simulink model "Md57StEnCtrl"  (R2018b)
settings: Solver=FixedStepDiscrete  StartTime=0.0  StopTime=10.0  FixedStep=0.01  RelTol=1e-3
undefined symbols (not defined in the file or in its folder): data, KeSMSuFirstRwStFwdBkwdPosDelta_Val, KeSMSw4SSecRwLtStLgrstUpwdDnwdOpenPos1_Val, PassStBkReclnEn_Clear, PassStBkReclnEn_Set, PassStFldEn_Clear, PassStFldEn_Set, PassStFwdBkwdEn_Clear, PassStFwdBkwdEn_Set, SecRwRtStBkReclnEn_Clear, SecRwRtStBkReclnEn_Set, SecRwRtStFwdBkwdEn_Clear, SecRwRtStFwdBkwdEn_Set, SecRwRtStLgrstInwdOtwdEn_Clear, SecRwRtStLgrstInwdOtwdEn_Set, SecRwRtStLgrstUpwdDnwdEn_Clear, SecRwRtStLgrstUpwdDnwdEn_Set, ThdRwLtStBkReclnEn_Clear, ThdRwLtStBkReclnEn_Set, ThdRwLtStFwdBkwdEn_Clear, ThdRwLtStFwdBkwdEn_Set, ThdRwRtStBkReclnEn_Clear, ThdRwRtStBkReclnEn_Set, ThdRwRtStFwdBkwdEn_Clear, ThdRwRtStFwdBkwdEn_Set, ZeroREn_Clear, ZeroREn_Set
libraries: simulink x1
(part 1 of 2)
settings Model: Creator=sn2xws  LastModifiedBy=sn2xws
settings Model: ModifiedHistory=|
  | 2024.10.15 V3.0.0 新增模式Md57
  | 2024.11.18 V3.0.1 CR946373
settings DataIOCC: SaveFormat=StructureWithTime
settings OptimizationCC: DefaultParameterBehavior=Inlined  EnhancedBackFolding=on  PassReuseOutputArgsAs=Individual arguments  ZeroExternalMemoryAtStartup=off  ZeroInternalMemoryAtStartup=off  OptimizeBlockOrder=speed  DifferentSizesBufferReuse=on  OptimizationCustomize=off
settings DebuggingCC: ParameterTunabilityLossMsg=error
settings SFSimCC: MATLABDynamicMemAlloc=off
settings RTWCC: SystemTargetFile=autosar.tlc  GenCodeOnly=on  TemplateMakefile=ert_default_tmf  Description=AUTOSAR  GenerateReport=on  IncludeHyperlinkInReport=on  LaunchReport=on  GenerateTraceInfo=on  GenerateTraceReport=on  GenerateTraceReportSl=on  GenerateTraceReportSf=on  GenerateTraceReportEml=on
settings CodeAppCC: ForceParamTrailComments=on  IgnoreCustomStorageClasses=off  OperatorAnnotations=on  SimulinkDataObjDesc=on  SFDataObjDesc=on  InsertBlockDesc=on
settings STFCustomTargetCC: TargetLangStandard=C99 (ISO)  MultiwordLength=256  ParMdlRefBuildCompliant=on  CompOptLevelCompliant=on  IncludeMdlTerminateFcn=off  CombineOutputUpdateFcns=on  SuppressErrorStatus=on  ERTCustomFileBanners=on  SupportNonFinite=off  SupportComplex=off  SupportContinuousTime=off  SupportNonInlinedSFcns=off  RemoveResetFunc=on  MATLABClassNameForMDSCustomization=Simulink.SoftwareTarget.ERTCustomization  AutosarCompliant=on  UseToolchainInfoCompliant=on  LookupTableObjectStructAxisOrder=2,1,3,4,...  LUTObjectStructOrderEvenSpacing=Size,Table,Breakpoints  SystemTargetFile=autosar.tlc
settings ERTTargetCC: TargetLangStandard=C99 (ISO)  ConcurrentExecutionCompliant=off  IncludeMdlTerminateFcn=off  SuppressErrorStatus=on  SupportNonFinite=off  SupportComplex=off  ModelStepFunctionPrototypeControlCompliant=off  CPPClassGenCompliant=off  AutosarCompliant=on  LookupTableObjectStructAxisOrder=2,1,3,4,...  LUTObjectStructOrderEvenSpacing=Size,Table,Breakpoints  InlinedParameterPlacement=NonHierarchical  ERTCustomFileTemplate=example_file_process.tlc  ERTFilePackagingFormat=Compact

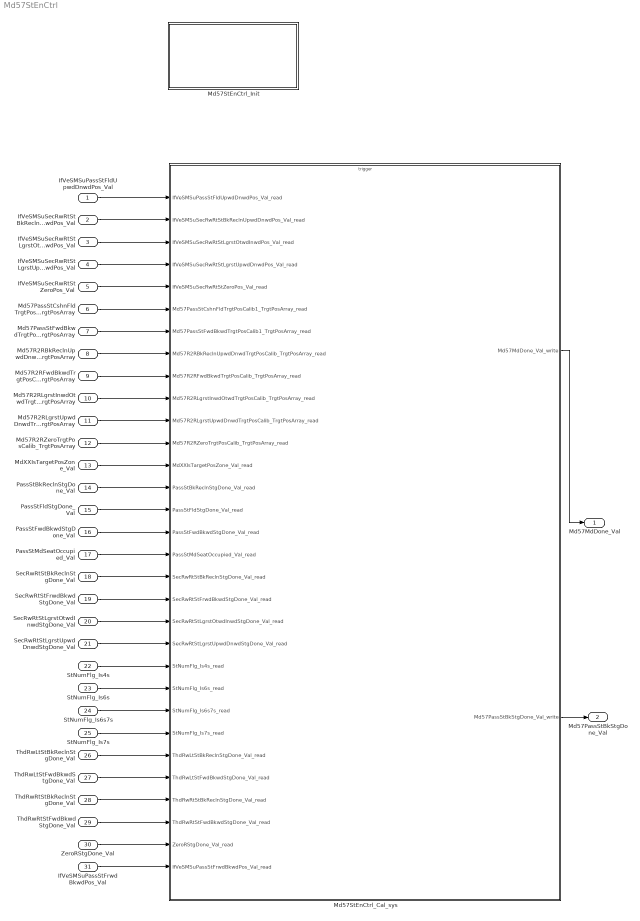
== system Md57StEnCtrl ==
  IfVeSMSuPassStFldUpwdDnwdPos_Val : Inport  OutDataTypeStr=uint16  PortDimensions=1
  IfVeSMSuSecRwRtStBkReclnUpwdDnwdPos_Val : Inport  Port=2  OutDataTypeStr=uint16  PortDimensions=1
  IfVeSMSuSecRwRtStLgrstOtwdInwdPos_Val : Inport  Port=3  OutDataTypeStr=uint16  PortDimensions=1
  IfVeSMSuSecRwRtStLgrstUpwdDnwdPos_Val : Inport  Port=4  OutDataTypeStr=uint16  PortDimensions=1
  IfVeSMSuSecRwRtStZeroPos_Val : Inport  Port=5  OutDataTypeStr=uint16  PortDimensions=1
  Md57PassStCshnFldTrgtPosCalib1_TrgtPosArray : Inport  Description=|  Port=6  OutDataTypeStr=uint16  PortDimensions=3
      | 0:Pos
      | 1:Max
      | 2:Min
  Md57PassStFwdBkwdTrgtPosCalib1_TrgtPosArray : Inport  Description=|  Port=7  OutDataTypeStr=uint16  PortDimensions=3
      | 0:Pos
      | 1:Max
      | 2:Min
  Md57R2RBkReclnUpwdDnwdTrgtPosCalib_TrgtPosArray : Inport  Description=|  Port=8  OutDataTypeStr=uint16  PortDimensions=3
      | 0:Pos
      | 1:Max
      | 2:Min
  Md57R2RFwdBkwdTrgtPosCalib_TrgtPosArray : Inport  Description=|  Port=9  OutDataTypeStr=uint16  PortDimensions=3
      | 0:Pos
      | 1:Max
      | 2:Min
  Md57R2RLgrstInwdOtwdTrgtPosCalib_TrgtPosArray : Inport  Description=|  Port=10  OutDataTypeStr=uint16  PortDimensions=3
      | 0:Pos
      | 1:Max
      | 2:Min
  Md57R2RLgrstUpwdDnwdTrgtPosCalib_TrgtPosArray : Inport  Description=|  Port=11  OutDataTypeStr=uint16  PortDimensions=3
      | 0:Pos
      | 1:Max
      | 2:Min
  Md57R2RZeroTrgtPosCalib_TrgtPosArray : Inport  Description=|  Port=12  OutDataTypeStr=uint16  PortDimensions=3
      | 0:Pos
      | 1:Max
      | 2:Min
  MdXXIsTargetPosZone_Val : Inport  Port=13  OutDataTypeStr=uint32  PortDimensions=1
  PassStBkReclnStgDone_Val : Inport  Port=14  OutDataTypeStr=boolean  PortDimensions=1
  PassStFldStgDone_Val : Inport  Port=15  OutDataTypeStr=boolean  PortDimensions=1
  PassStFwdBkwdStgDone_Val : Inport  Port=16  OutDataTypeStr=boolean  PortDimensions=1
  PassStMdSeatOccupied_Val : Inport  Port=17  OutDataTypeStr=boolean  PortDimensions=1
  SecRwRtStBkReclnStgDone_Val : Inport  Port=18  OutDataTypeStr=boolean  PortDimensions=1
  SecRwRtStFrwdBkwdStgDone_Val : Inport  Port=19  OutDataTypeStr=boolean  PortDimensions=1
  SecRwRtStLgrstOtwdInwdStgDone_Val : Inport  Port=20  OutDataTypeStr=boolean  PortDimensions=1
  SecRwRtStLgrstUpwdDnwdStgDone_Val : Inport  Port=21  OutDataTypeStr=boolean  PortDimensions=1
  StNumFlg_Is4s : Inport  Port=22  OutDataTypeStr=boolean  PortDimensions=1
  StNumFlg_Is6s : Inport  Port=23  OutDataTypeStr=boolean  PortDimensions=1
  StNumFlg_Is6s7s : Inport  Port=24  OutDataTypeStr=boolean  PortDimensions=1
  StNumFlg_Is7s : Inport  Port=25  OutDataTypeStr=boolean  PortDimensions=1
  ThdRwLtStBkReclnStgDone_Val : Inport  Port=26  OutDataTypeStr=boolean  PortDimensions=1
  ThdRwLtStFwdBkwdStgDone_Val : Inport  Port=27  OutDataTypeStr=boolean  PortDimensions=1
  ThdRwRtStBkReclnStgDone_Val : Inport  Port=28  OutDataTypeStr=boolean  PortDimensions=1
  ThdRwRtStFwdBkwdStgDone_Val : Inport  Port=29  OutDataTypeStr=boolean  PortDimensions=1
  ZeroRStgDone_Val : Inport  Port=30  OutDataTypeStr=boolean  PortDimensions=1
  IfVeSMSuPassStFrwdBkwdPos_Val : Inport  Port=31  OutDataTypeStr=uint16  PortDimensions=1
  Md57StEnCtrl_Cal_sys : Subsystem
  Md57StEnCtrl_Init : Subsystem
  Md57MdDone_Val : Outport  OutDataTypeStr=uint8  PortDimensions=1
  Md57PassStBkStgDone_Val : Outport  Port=2  OutDataTypeStr=boolean  PortDimensions=1
  wires:
  IfVeSMSuPassStFldUpwdDnwdPos_Val/1 -> Md57StEnCtrl_Cal_sys/1(IfVeSMSuPassStFldUpwdDnwdPos_Val_read)
  IfVeSMSuSecRwRtStBkReclnUpwdDnwdPos_Val/1 -> Md57StEnCtrl_Cal_sys/2(IfVeSMSuSecRwRtStBkReclnUpwdDnwdPos_Val_read)
  IfVeSMSuSecRwRtStLgrstOtwdInwdPos_Val/1 -> Md57StEnCtrl_Cal_sys/3(IfVeSMSuSecRwRtStLgrstOtwdInwdPos_Val_read)
  IfVeSMSuSecRwRtStLgrstUpwdDnwdPos_Val/1 -> Md57StEnCtrl_Cal_sys/4(IfVeSMSuSecRwRtStLgrstUpwdDnwdPos_Val_read)
  IfVeSMSuSecRwRtStZeroPos_Val/1 -> Md57StEnCtrl_Cal_sys/5(IfVeSMSuSecRwRtStZeroPos_Val_read)
  Md57PassStCshnFldTrgtPosCalib1_TrgtPosArray/1 -> Md57StEnCtrl_Cal_sys/6(Md57PassStCshnFldTrgtPosCalib1_TrgtPosArray_read)
  Md57PassStFwdBkwdTrgtPosCalib1_TrgtPosArray/1 -> Md57StEnCtrl_Cal_sys/7(Md57PassStFwdBkwdTrgtPosCalib1_TrgtPosArray_read)
  Md57R2RBkReclnUpwdDnwdTrgtPosCalib_TrgtPosArray/1 -> Md57StEnCtrl_Cal_sys/8(Md57R2RBkReclnUpwdDnwdTrgtPosCalib_TrgtPosArray_read)
  Md57R2RFwdBkwdTrgtPosCalib_TrgtPosArray/1 -> Md57StEnCtrl_Cal_sys/9(Md57R2RFwdBkwdTrgtPosCalib_TrgtPosArray_read)
  Md57R2RLgrstInwdOtwdTrgtPosCalib_TrgtPosArray/1 -> Md57StEnCtrl_Cal_sys/10(Md57R2RLgrstInwdOtwdTrgtPosCalib_TrgtPosArray_read)
  Md57R2RLgrstUpwdDnwdTrgtPosCalib_TrgtPosArray/1 -> Md57StEnCtrl_Cal_sys/11(Md57R2RLgrstUpwdDnwdTrgtPosCalib_TrgtPosArray_read)
  Md57R2RZeroTrgtPosCalib_TrgtPosArray/1 -> Md57StEnCtrl_Cal_sys/12(Md57R2RZeroTrgtPosCalib_TrgtPosArray_read)
  MdXXIsTargetPosZone_Val/1 -> Md57StEnCtrl_Cal_sys/13(MdXXIsTargetPosZone_Val_read)
  PassStBkReclnStgDone_Val/1 -> Md57StEnCtrl_Cal_sys/14(PassStBkReclnStgDone_Val_read)
  PassStFldStgDone_Val/1 -> Md57StEnCtrl_Cal_sys/15(PassStFldStgDone_Val_read)
  PassStFwdBkwdStgDone_Val/1 -> Md57StEnCtrl_Cal_sys/16(PassStFwdBkwdStgDone_Val_read)
  PassStMdSeatOccupied_Val/1 -> Md57StEnCtrl_Cal_sys/17(PassStMdSeatOccupied_Val_read)
  SecRwRtStBkReclnStgDone_Val/1 -> Md57StEnCtrl_Cal_sys/18(SecRwRtStBkReclnStgDone_Val_read)
  SecRwRtStFrwdBkwdStgDone_Val/1 -> Md57StEnCtrl_Cal_sys/19(SecRwRtStFrwdBkwdStgDone_Val_read)
  SecRwRtStLgrstOtwdInwdStgDone_Val/1 -> Md57StEnCtrl_Cal_sys/20(SecRwRtStLgrstOtwdInwdStgDone_Val_read)
  SecRwRtStLgrstUpwdDnwdStgDone_Val/1 -> Md57StEnCtrl_Cal_sys/21(SecRwRtStLgrstUpwdDnwdStgDone_Val_read)
  StNumFlg_Is4s/1 -> Md57StEnCtrl_Cal_sys/22(StNumFlg_Is4s_read)
  StNumFlg_Is6s/1 -> Md57StEnCtrl_Cal_sys/23(StNumFlg_Is6s_read)
  StNumFlg_Is6s7s/1 -> Md57StEnCtrl_Cal_sys/24(StNumFlg_Is6s7s_read)
  StNumFlg_Is7s/1 -> Md57StEnCtrl_Cal_sys/25(StNumFlg_Is7s_read)
  ThdRwLtStBkReclnStgDone_Val/1 -> Md57StEnCtrl_Cal_sys/26(ThdRwLtStBkReclnStgDone_Val_read)
  ThdRwLtStFwdBkwdStgDone_Val/1 -> Md57StEnCtrl_Cal_sys/27(ThdRwLtStFwdBkwdStgDone_Val_read)
  ThdRwRtStBkReclnStgDone_Val/1 -> Md57StEnCtrl_Cal_sys/28(ThdRwRtStBkReclnStgDone_Val_read)
  ThdRwRtStFwdBkwdStgDone_Val/1 -> Md57StEnCtrl_Cal_sys/29(ThdRwRtStFwdBkwdStgDone_Val_read)
  ZeroRStgDone_Val/1 -> Md57StEnCtrl_Cal_sys/30(ZeroRStgDone_Val_read)
  Md57StEnCtrl_Cal_sys/1(Md57MdDone_Val_write) -> Md57MdDone_Val/1
  IfVeSMSuPassStFrwdBkwdPos_Val/1 -> Md57StEnCtrl_Cal_sys/31(IfVeSMSuPassStFrwdBkwdPos_Val_read)
  Md57StEnCtrl_Cal_sys/2(Md57PassStBkStgDone_Val_write) -> Md57PassStBkStgDone_Val/1

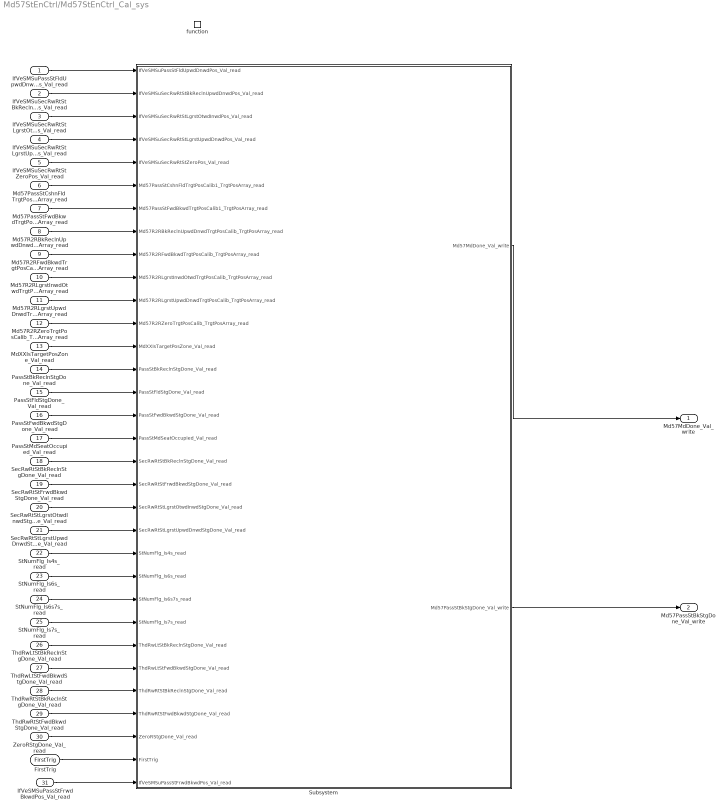
== system Md57StEnCtrl/Md57StEnCtrl_Cal_sys ==
  IfVeSMSuPassStFldUpwdDnwdPos_Val_read : Inport
  IfVeSMSuSecRwRtStBkReclnUpwdDnwdPos_Val_read : Inport  Port=2
  IfVeSMSuSecRwRtStLgrstOtwdInwdPos_Val_read : Inport  Port=3
  IfVeSMSuSecRwRtStLgrstUpwdDnwdPos_Val_read : Inport  Port=4
  IfVeSMSuSecRwRtStZeroPos_Val_read : Inport  Port=5
  Md57PassStCshnFldTrgtPosCalib1_TrgtPosArray_read : Inport  Port=6
  Md57PassStFwdBkwdTrgtPosCalib1_TrgtPosArray_read : Inport  Port=7
  Md57R2RBkReclnUpwdDnwdTrgtPosCalib_TrgtPosArray_read : Inport  Port=8
  Md57R2RFwdBkwdTrgtPosCalib_TrgtPosArray_read : Inport  Port=9
  Md57R2RLgrstInwdOtwdTrgtPosCalib_TrgtPosArray_read : Inport  Port=10
  Md57R2RLgrstUpwdDnwdTrgtPosCalib_TrgtPosArray_read : Inport  Port=11
  Md57R2RZeroTrgtPosCalib_TrgtPosArray_read : Inport  Port=12
  MdXXIsTargetPosZone_Val_read : Inport  Port=13
  PassStBkReclnStgDone_Val_read : Inport  Port=14
  PassStFldStgDone_Val_read : Inport  Port=15
  PassStFwdBkwdStgDone_Val_read : Inport  Port=16
  PassStMdSeatOccupied_Val_read : Inport  Port=17
  SecRwRtStBkReclnStgDone_Val_read : Inport  Port=18
  SecRwRtStFrwdBkwdStgDone_Val_read : Inport  Port=19
  SecRwRtStLgrstOtwdInwdStgDone_Val_read : Inport  Port=20
  SecRwRtStLgrstUpwdDnwdStgDone_Val_read : Inport  Port=21
  StNumFlg_Is4s_read : Inport  Port=22
  StNumFlg_Is6s_read : Inport  Port=23
  StNumFlg_Is6s7s_read : Inport  Port=24
  StNumFlg_Is7s_read : Inport  Port=25
  ThdRwLtStBkReclnStgDone_Val_read : Inport  Port=26
  ThdRwLtStFwdBkwdStgDone_Val_read : Inport  Port=27
  ThdRwRtStBkReclnStgDone_Val_read : Inport  Port=28
  ThdRwRtStFwdBkwdStgDone_Val_read : Inport  Port=29
  ZeroRStgDone_Val_read : Inport  Port=30
  IfVeSMSuPassStFrwdBkwdPos_Val_read : Inport  Port=31
  function : TriggerPort  TriggerType=function-call  IsSimulinkFunction=on  FunctionName=Md57StEnCtrl_Cal  VariantControl=(inherit)
  Subsystem : Subsystem
  FirstTrig : ArgIn  OutDataTypeStr=boolean  ArgumentName=FirstTrig
  Md57MdDone_Val_write : Outport
      settings: EnsureOutportIsVirtual=on
  Md57PassStBkStgDone_Val_write : Outport  Port=2
      settings: EnsureOutportIsVirtual=on
  wires:
  IfVeSMSuPassStFldUpwdDnwdPos_Val_read/1 -> Subsystem/1(IfVeSMSuPassStFldUpwdDnwdPos_Val_read)
  IfVeSMSuSecRwRtStBkReclnUpwdDnwdPos_Val_read/1 -> Subsystem/2(IfVeSMSuSecRwRtStBkReclnUpwdDnwdPos_Val_read)
  IfVeSMSuSecRwRtStLgrstOtwdInwdPos_Val_read/1 -> Subsystem/3(IfVeSMSuSecRwRtStLgrstOtwdInwdPos_Val_read)
  IfVeSMSuSecRwRtStLgrstUpwdDnwdPos_Val_read/1 -> Subsystem/4(IfVeSMSuSecRwRtStLgrstUpwdDnwdPos_Val_read)
  IfVeSMSuSecRwRtStZeroPos_Val_read/1 -> Subsystem/5(IfVeSMSuSecRwRtStZeroPos_Val_read)
  Md57PassStCshnFldTrgtPosCalib1_TrgtPosArray_read/1 -> Subsystem/6(Md57PassStCshnFldTrgtPosCalib1_TrgtPosArray_read)
  Md57PassStFwdBkwdTrgtPosCalib1_TrgtPosArray_read/1 -> Subsystem/7(Md57PassStFwdBkwdTrgtPosCalib1_TrgtPosArray_read)
  Md57R2RBkReclnUpwdDnwdTrgtPosCalib_TrgtPosArray_read/1 -> Subsystem/8(Md57R2RBkReclnUpwdDnwdTrgtPosCalib_TrgtPosArray_read)
  Md57R2RFwdBkwdTrgtPosCalib_TrgtPosArray_read/1 -> Subsystem/9(Md57R2RFwdBkwdTrgtPosCalib_TrgtPosArray_read)
  Md57R2RLgrstInwdOtwdTrgtPosCalib_TrgtPosArray_read/1 -> Subsystem/10(Md57R2RLgrstInwdOtwdTrgtPosCalib_TrgtPosArray_read)
  Md57R2RLgrstUpwdDnwdTrgtPosCalib_TrgtPosArray_read/1 -> Subsystem/11(Md57R2RLgrstUpwdDnwdTrgtPosCalib_TrgtPosArray_read)
  Md57R2RZeroTrgtPosCalib_TrgtPosArray_read/1 -> Subsystem/12(Md57R2RZeroTrgtPosCalib_TrgtPosArray_read)
  MdXXIsTargetPosZone_Val_read/1 -> Subsystem/13(MdXXIsTargetPosZone_Val_read)
  PassStBkReclnStgDone_Val_read/1 -> Subsystem/14(PassStBkReclnStgDone_Val_read)
  PassStFldStgDone_Val_read/1 -> Subsystem/15(PassStFldStgDone_Val_read)
  PassStFwdBkwdStgDone_Val_read/1 -> Subsystem/16(PassStFwdBkwdStgDone_Val_read)
  PassStMdSeatOccupied_Val_read/1 -> Subsystem/17(PassStMdSeatOccupied_Val_read)
  SecRwRtStBkReclnStgDone_Val_read/1 -> Subsystem/18(SecRwRtStBkReclnStgDone_Val_read)
  SecRwRtStFrwdBkwdStgDone_Val_read/1 -> Subsystem/19(SecRwRtStFrwdBkwdStgDone_Val_read)
  SecRwRtStLgrstOtwdInwdStgDone_Val_read/1 -> Subsystem/20(SecRwRtStLgrstOtwdInwdStgDone_Val_read)
  SecRwRtStLgrstUpwdDnwdStgDone_Val_read/1 -> Subsystem/21(SecRwRtStLgrstUpwdDnwdStgDone_Val_read)
  StNumFlg_Is4s_read/1 -> Subsystem/22(StNumFlg_Is4s_read)
  StNumFlg_Is6s_read/1 -> Subsystem/23(StNumFlg_Is6s_read)
  StNumFlg_Is6s7s_read/1 -> Subsystem/24(StNumFlg_Is6s7s_read)
  StNumFlg_Is7s_read/1 -> Subsystem/25(StNumFlg_Is7s_read)
  ThdRwLtStBkReclnStgDone_Val_read/1 -> Subsystem/26(ThdRwLtStBkReclnStgDone_Val_read)
  ThdRwLtStFwdBkwdStgDone_Val_read/1 -> Subsystem/27(ThdRwLtStFwdBkwdStgDone_Val_read)
  ThdRwRtStBkReclnStgDone_Val_read/1 -> Subsystem/28(ThdRwRtStBkReclnStgDone_Val_read)
  ThdRwRtStFwdBkwdStgDone_Val_read/1 -> Subsystem/29(ThdRwRtStFwdBkwdStgDone_Val_read)
  ZeroRStgDone_Val_read/1 -> Subsystem/30(ZeroRStgDone_Val_read)
  Subsystem/1(Md57MdDone_Val_write) -> Md57MdDone_Val_write/1
  FirstTrig/1 -> Subsystem/31(FirstTrig)
  IfVeSMSuPassStFrwdBkwdPos_Val_read/1 -> Subsystem/32(IfVeSMSuPassStFrwdBkwdPos_Val_read)
  Subsystem/2(Md57PassStBkStgDone_Val_write) -> Md57PassStBkStgDone_Val_write/1

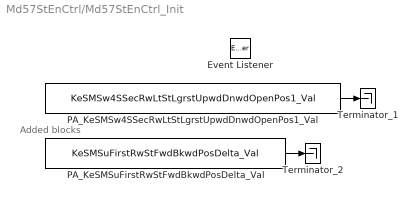
== system Md57StEnCtrl/Md57StEnCtrl_Init ==
  note: Added blocks
  Event Listener : EventListener  EventName=reset
  PA_KeSMSuFirstRwStFwdBkwdPosDelta_Val : Constant  Value=KeSMSuFirstRwStFwdBkwdPosDelta_Val
  PA_KeSMSw4SSecRwLtStLgrstUpwdDnwdOpenPos1_Val : Constant  Value=KeSMSw4SSecRwLtStLgrstUpwdDnwdOpenPos1_Val
  Terminator_1 : Terminator
  Terminator_2 : Terminator
  wires:
  PA_KeSMSw4SSecRwLtStLgrstUpwdDnwdOpenPos1_Val/1 -> Terminator_1/1
  PA_KeSMSuFirstRwStFwdBkwdPosDelta_Val/1 -> Terminator_2/1

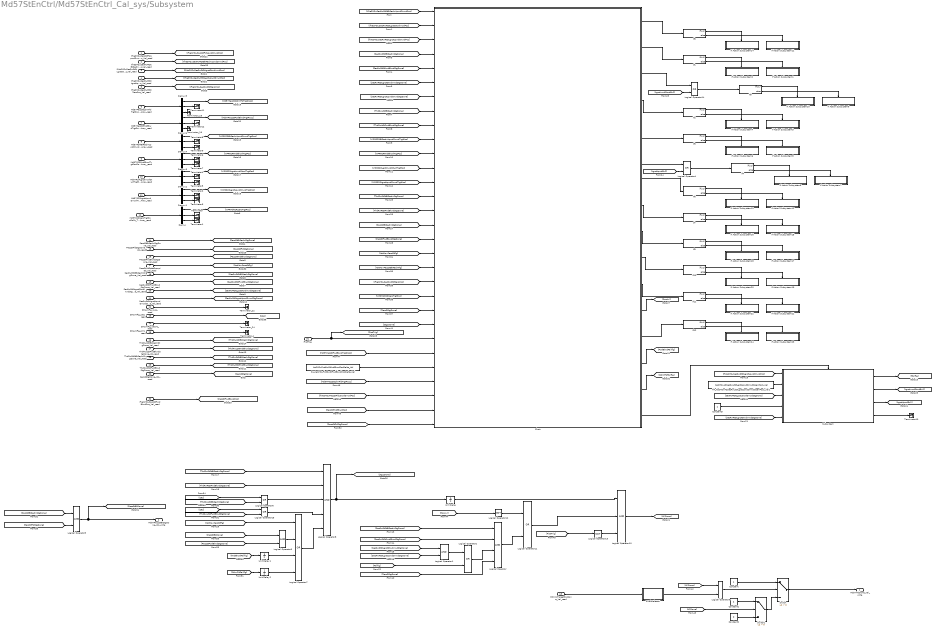
== system Md57StEnCtrl/Md57StEnCtrl_Cal_sys/Subsystem ==
  IfVeSMSuPassStFldUpwdDnwdPos_Val_read : Inport
  IfVeSMSuSecRwRtStBkReclnUpwdDnwdPos_Val_read : Inport  Port=2
  IfVeSMSuSecRwRtStLgrstOtwdInwdPos_Val_read : Inport  Port=3
  IfVeSMSuSecRwRtStLgrstUpwdDnwdPos_Val_read : Inport  Port=4
  IfVeSMSuSecRwRtStZeroPos_Val_read : Inport  Port=5
  Md57PassStCshnFldTrgtPosCalib1_TrgtPosArray_read : Inport  Port=6
  Md57PassStFwdBkwdTrgtPosCalib1_TrgtPosArray_read : Inport  Port=7
  Md57R2RBkReclnUpwdDnwdTrgtPosCalib_TrgtPosArray_read : Inport  Port=8
  Md57R2RFwdBkwdTrgtPosCalib_TrgtPosArray_read : Inport  Port=9
  Md57R2RLgrstInwdOtwdTrgtPosCalib_TrgtPosArray_read : Inport  Port=10
  Md57R2RLgrstUpwdDnwdTrgtPosCalib_TrgtPosArray_read : Inport  Port=11
  Md57R2RZeroTrgtPosCalib_TrgtPosArray_read : Inport  Port=12
  MdXXIsTargetPosZone_Val_read : Inport  Port=13
  PassStBkReclnStgDone_Val_read : Inport  Port=14
  PassStFldStgDone_Val_read : Inport  Port=15
  PassStFwdBkwdStgDone_Val_read : Inport  Port=16
  PassStMdSeatOccupied_Val_read : Inport  Port=17
  SecRwRtStBkReclnStgDone_Val_read : Inport  Port=18
  SecRwRtStFrwdBkwdStgDone_Val_read : Inport  Port=19
  SecRwRtStLgrstOtwdInwdStgDone_Val_read : Inport  Port=20
  SecRwRtStLgrstUpwdDnwdStgDone_Val_read : Inport  Port=21
  StNumFlg_Is4s_read : Inport  Port=22
  StNumFlg_Is6s_read : Inport  Port=23
  StNumFlg_Is6s7s_read : Inport  Port=24
  StNumFlg_Is7s_read : Inport  Port=25
  ThdRwLtStBkReclnStgDone_Val_read : Inport  Port=26
  ThdRwLtStFwdBkwdStgDone_Val_read : Inport  Port=27
  ThdRwRtStBkReclnStgDone_Val_read : Inport  Port=28
  ThdRwRtStFwdBkwdStgDone_Val_read : Inport  Port=29
  ZeroRStgDone_Val_read : Inport  Port=30
  FirstTrig : Inport  Port=31
  IfVeSMSuPassStFrwdBkwdPos_Val_read : Inport  Port=32
  32BitSelector : Subsystem  mask(32 Bit Selector){BitNum=20}
      mask prompts: BitNum "Select Bit Number"
      mask help: Allows selection of a particular bit (0-31) out of a packed word up to 32 bits long. Output will be true if the bit number selected via the mask parameter is equal to one.
      mask TypeOptions BitNum: 0 | 1 | 2 | 3 | 4 | 5 | 6 | 7 | 8 | 9 | 10 | 11 | 12 | 13 | 14 | 15 | 16 | 17 | 18 | 19 | 20 | 21 | 22 | 23 | 24 | 25 | 26 | 27 | 28 | 29 | 30 | 31
      mask Display:
      | text(0.5, 0.8,'BIT','horizontalAlignment','center')
      | text(0.5, 0.5,'SELECTOR','horizontalAlignment','center')
      | text(0.5, 0.2,['-- Bit ',char(get_param(gcb,'BitNum')),' --'],'horizontalAlignment','center')
  Chart : Stateflow chart  TreatAsAtomicUnit=on
  Constant : Constant  OutDataTypeStr=uint8
  Constant1 : Constant  Value=2  OutDataTypeStr=uint8
  Constant2 : Constant  Value=0  OutDataTypeStr=uint8
  Constant3 : Constant  OutDataTypeStr=boolean
  Demux{,1..6} (7 alike) : Demux  Outputs=3
  If Action Subsystem1 : Subsystem  TreatAsAtomicUnit=on
  If Action Subsystem10 : Subsystem  TreatAsAtomicUnit=on
  If Action Subsystem11 : Subsystem  TreatAsAtomicUnit=on
  If Action Subsystem12 : Subsystem  TreatAsAtomicUnit=on
  If Action Subsystem13 : Subsystem  TreatAsAtomicUnit=on
  If Action Subsystem14 : Subsystem  TreatAsAtomicUnit=on
  If Action Subsystem15 : Subsystem  TreatAsAtomicUnit=on
  If Action Subsystem16 : Subsystem  TreatAsAtomicUnit=on
  If Action Subsystem17 : Subsystem  TreatAsAtomicUnit=on
  If Action Subsystem18 : Subsystem  TreatAsAtomicUnit=on
  If Action Subsystem19 : Subsystem  TreatAsAtomicUnit=on
  If Action Subsystem2 : Subsystem  TreatAsAtomicUnit=on
  If Action Subsystem20 : Subsystem  TreatAsAtomicUnit=on
  If Action Subsystem21 : Subsystem  TreatAsAtomicUnit=on
  If Action Subsystem22 : Subsystem  TreatAsAtomicUnit=on
  If Action Subsystem23 : Subsystem  TreatAsAtomicUnit=on
  If Action Subsystem24 : Subsystem  TreatAsAtomicUnit=on
  If Action Subsystem3 : Subsystem  TreatAsAtomicUnit=on
  If Action Subsystem4 : Subsystem  TreatAsAtomicUnit=on
  If Action Subsystem5 : Subsystem  TreatAsAtomicUnit=on
  If Action Subsystem6 : Subsystem  TreatAsAtomicUnit=on
  If Action Subsystem7 : Subsystem  TreatAsAtomicUnit=on
  If Action Subsystem8 : Subsystem  TreatAsAtomicUnit=on
  If Action Subsystem9 : Subsystem  TreatAsAtomicUnit=on
  If{1..12} (12 alike) : If  IfExpression=u1
  Logical Operator : Logic  Inputs=4  AllPortsSameDT=off  OutDataTypeStr=boolean
  Logical Operator{1,3,5,9} (4 alike) : Logic  AllPortsSameDT=off  OutDataTypeStr=boolean
  Logical Operator10 : Logic  Inputs=3  AllPortsSameDT=off  OutDataTypeStr=boolean
  Logical Operator{2,4,6,11,14..15} (6 alike) : Logic  Operator=OR  AllPortsSameDT=off  OutDataTypeStr=boolean
  Logical Operator12 : Logic  Operator=NOT  AllPortsSameDT=off  OutDataTypeStr=boolean
  Logical Operator13 : Logic  Operator=NOT  AllPortsSameDT=off  OutDataTypeStr=boolean
  Logical Operator7 : Logic  Operator=OR  Inputs=4  AllPortsSameDT=off  OutDataTypeStr=boolean
  Logical Operator8 : Logic  Inputs=5  AllPortsSameDT=off  OutDataTypeStr=boolean
  PA_KeSMSuFirstRwStFwdBkwdPosDelta_Val : Constant  Value=KeSMSuFirstRwStFwdBkwdPosDelta_Val
  PA_KeSMSw4SSecRwLtStLgrstUpwdDnwdOpenPos1_Val1 : Constant  Value=KeSMSw4SSecRwLtStLgrstUpwdDnwdOpenPos1_Val
  Subsystem : Subsystem
  Switch : Switch  Criteria=u2 > Threshold
  Switch1 : Switch  Criteria=u2 > Threshold
  Terminator{,1..12} (13 alike) : Terminator
  Terminator_{1,18..19,22,24} (5 alike) : Terminator
  Unit Delay : UnitDelay  SampleTime=-1
  Unit Delay1 : UnitDelay  SampleTime=-1
  Unit Delay2 : UnitDelay  SampleTime=-1
  Md57MdDone_Val_write : Outport
      settings: EnsureOutportIsVirtual=on
  Md57PassStBkStgDone_Val_write : Outport  Port=2
      settings: EnsureOutportIsVirtual=on
  wires:
  ThdRwLtStBkReclnStgDone_Val_read/1 -> [ThdRwLtStBkReclnStgDone]
  StNumFlg_Is4s_read/1 -> Terminator_22/1
  PassStFwdBkwdStgDone_Val_read/1 -> [PassStFwdBkwdStgDone]
  ThdRwRtStBkReclnStgDone_Val_read/1 -> [ThdRwRtStBkReclnStgDone]
  SecRwRtStLgrstUpwdDnwdStgDone_Val_read/1 -> [SecRwRtStLgrstUpwdDnwdStgDone]
  ThdRwLtStFwdBkwdStgDone_Val_read/1 -> [ThdRwLtStFwdBkwdStgDone]
  StNumFlg_Is6s_read/1 -> [Is6s]
  ZeroRStgDone_Val_read/1 -> [ZeroRStgDone]
  PassStMdSeatOccupied_Val_read/1 -> [NotMovPassStFlg]
  SecRwRtStFrwdBkwdStgDone_Val_read/1 -> [SecRwRtStFrwdBkwdStgDone]
  SecRwRtStLgrstOtwdInwdStgDone_Val_read/1 -> [SecRwRtStLgrstOtwdInwdStgDone]
  PassStBkReclnStgDone_Val_read/1 -> [PassStBkReclnStgDone]
  PassStFldStgDone_Val_read/1 -> [PassStFldStgDone]
  SecRwRtStBkReclnStgDone_Val_read/1 -> [SecRwRtStBkReclnStgDone]
  StNumFlg_Is6s7s_read/1 -> Terminator_24/1
  StNumFlg_Is7s_read/1 -> Terminator_1/1
  ThdRwRtStFwdBkwdStgDone_Val_read/1 -> [ThdRwRtStFwdBkwdStgDone]
  [AllDone] -> Switch1/2
  MdXXIsTargetPosZone_Val_read/1 -> 32BitSelector/1(x)
  Constant1/1 -> Switch1/1
  Logical Operator9/1 -> Switch/2
  32BitSelector/1(y) -> Logical Operator9/2
  Constant/1 -> Switch/1
  Switch/1 -> Md57MdDone_Val_write/1
  Constant2/1 -> Switch1/3
  [AllDone] -> Logical Operator9/1
  Switch1/1 -> Switch/3
  Logical Operator11/1 -> Logical Operator10/2
  [FirstTrig] -> Logical Operator13/1
  [ZeroRStgDone] -> Logical Operator/4
  Logical Operator8/1 -> [Stg1Done], Unit Delay/1
  [SecRwRtStLgrstOtwdInwdStgDone] -> Logical Operator1/1
  Logical Operator/1 -> Logical Operator11/2
  Logical Operator12/1 -> Logical Operator11/1
  [SecRwRtStFrwdBkwdStgDone] -> Logical Operator/2
  Logical Operator13/1 -> Logical Operator10/3
  [PosAvl] -> Logical Operator12/1
  [Failflg] -> Logical Operator2/2
  Logical Operator10/1 -> [AllDone]
  Logical Operator7/1 -> Logical Operator8/5
  Logical Operator5/1 -> Logical Operator7/2
  [ThdRwRtStBkReclnStgDone] -> Logical Operator8/1
  [ThdRwRtStFwdBkwdStgDone] -> Logical Operator8/2
  [SecRwRtStLgrstUpwdDnwdStgDone] -> Logical Operator1/2
  Logical Operator2/1 -> Logical Operator/3
  Logical Operator1/1 -> Logical Operator2/1
  Unit Delay/1 -> Logical Operator10/1
  [NotMovPassStFlg] -> Logical Operator7/1
  [SecRwRtStBkReclnStgDone] -> Logical Operator/1
  [PassStFwdBkwdStgDone] -> Logical Operator5/2
  If3/2 -> If Action Subsystem5/Action
  [VIPRR2RBkReclnUpwdDnwdTrgtPos] -> Chart/10(VIPLR2LBkReclnUpwdDnwdTrgtPos)
  Chart/4(ThdRwLtStBkReclnEn) -> If2/1
  [LgrstInwdOtwdEn2] -> Logical Operator14/2
  [SecRwRtStLgrstUpwdDnwdStgDone] -> Chart/7(SecRwLtStLgrstUpwdDnwdStgDone)
  Subsystem/4(FtrstEn) -> Terminator10/1
  If4/1 -> If Action Subsystem8/Action
  If3/1 -> If Action Subsystem6/Action
  If6/2 -> If Action Subsystem12/Action
  Chart/16(LgrstOpn()) -> Subsystem/Trigger
  [NotMovPassStFlg] -> Chart/18(NotMovPassStFlg)
  If9/1 -> If Action Subsystem18/Action
  If1/1 -> If Action Subsystem2/Action
  Chart/6(SecRwLtStLgrstUpwdDnwdEn) -> Logical Operator4/1
  If5/1 -> If Action Subsystem10/Action
  [VIPRMdR2RZeroTrgtPos] -> Chart/21(VIPRMdR2RZeroTrgtPos)
  If1/2 -> If Action Subsystem1/Action
  [ThdRwLtStFwdBkwdStgDone] -> Chart/9(ThdRwLtStFwdBkwdStgDone)
  [IfVeSMSuSecRwRtStLgrstUpwdDnwdPos] -> Chart/3(IfVeSMSuSecRwLtStLgrstUpwdDnwdPos)
  If4/2 -> If Action Subsystem7/Action
  Chart/8(ThdRwRtStFwdBkwdEn) -> If7/1
  Chart/5(ThdRwLtStFwdBkwdEn) -> If3/1
  Chart/3(SecRwLtStLgrstOtwdInwdEn) -> Logical Operator14/1
  [ZeroRStgDone] -> Chart/22(ZeroRStgDone)
  PA_KeSMSw4SSecRwLtStLgrstUpwdDnwdOpenPos1_Val1/1 -> Subsystem/2(LgrstUpwdDnwdOpenPos1)
  If11/1 -> If Action Subsystem22/Action
  [IfVeSMSuSecRwRtStLgrstUpwdDnwdPos] -> Subsystem/1(LgrstUpwdDnwdPos)
  Logical Operator4/1 -> If4/1
  [PassStBkReclnStgDone] -> Chart/16(PassStBkReclnStgDone)
  Chart/12(PosAvl) -> [PosAvl]
  Subsystem/1(Failflg) -> [Failflg]
  [NotMovPassStBkReclnFlg] -> Chart/19(NotMovPassStBkReclnFlg)
  Chart/11(SecRwStZeroEn) -> If11/1
  If11/2 -> If Action Subsystem21/Action
  Chart/7(ThdRwRtStBkReclnEn) -> If6/1
  If8/2 -> If Action Subsystem11/Action
  [ThdRwRtStBkReclnStgDone] -> Chart/14(ThdRwRtStBkReclnStgDone)
  [Stg1Done] -> Chart/23(Stg1Done)
  Logical Operator14/1 -> If5/1
  [SecRwRtStFrwdBkwdStgDone] -> Chart/5(SecRwLtStFrwdBkwdStgDone)
  If10/2 -> If Action Subsystem19/Action
  [SecRwRtStLgrstUpwdDnwdStgDone] -> Subsystem/3(LgrstUpwdStgDone)
  Constant3/1 -> Subsystem/4(FtrstStgDone)
  [VIPRR2RFwdBkwdTrgtPos] -> Chart/11(VIPLR2LFwdBkwdTrgtPos)
  Chart/9(PassStBkReclnEn) -> If9/1
  [IfVeSMSuSecRwRtStBkReclnUpwdDnwdPos] -> Chart/1(IfVeSMSuSecRwLtStBkReclnUpwdDnwdPos)
  If2/1 -> If Action Subsystem4/Action
  Subsystem/3(LgrstUpwdDnwdEn) -> [LgrstUpwdEn2]
  Chart/10(PassStFwdBkwdEn) -> If10/1
  [SecRwRtStBkReclnStgDone] -> Chart/4(SecRwLtStBkReclnStgDone)
  [SecRwRtStLgrstOtwdInwdStgDone] -> Chart/6(SecRwLtStLgrstOtwdInwdStgDone)
  [LgrstUpwdEn2] -> Logical Operator4/2
  If5/2 -> If Action Subsystem9/Action
  If10/1 -> If Action Subsystem20/Action
  [SecRwRtStLgrstOtwdInwdStgDone] -> Subsystem/5(LgrstInwdStgDone)
  [ThdRwRtStFwdBkwdStgDone] -> Chart/15(ThdRwRtStFwdBkwdStgDone)
  Subsystem/2(LgrstInwdOtwdEn) -> [LgrstInwdOtwdEn2]
  [VIPRR2RLgrstInwdOtwdTrgtPos] -> Chart/12(VIPLR2LLgrstInwdOtwdTrgtPos)
  FirstTrig/1 -> [FirstTrig], Chart/24(FirstTrig)
  Chart/1(SecRwLtStBkReclnEn) -> If8/1
  If6/1 -> If Action Subsystem13/Action
  If2/2 -> If Action Subsystem3/Action
  If9/2 -> If Action Subsystem17/Action
  If7/1 -> If Action Subsystem16/Action
  [IfVeSMSuSecRwRtStLgrstOtwdInwdPos] -> Chart/2(IfVeSMSuSecRwLtStLgrstOtwdInwdPos)
  Chart/2(SecRwLtStFrwdBkwdEn) -> If1/1
  If8/1 -> If Action Subsystem14/Action
  If7/2 -> If Action Subsystem15/Action
  [VIPRR2RLgrstUpwdDnwdTrgtPos] -> Chart/13(VIPLR2LLgrstUpwdDnwdTrgtPos)
  [PassStFwdBkwdStgDone] -> Chart/17(PassStFwdBkwdStgDone)
  [IfVeSMSuSecRwRtStZeroPos] -> Chart/20(IfVeSMSuSecRwRtStZeroPos)
  [ThdRwLtStBkReclnStgDone] -> Chart/8(ThdRwLtStBkReclnStgDone)
  IfVeSMSuSecRwRtStLgrstOtwdInwdPos_Val_read/1 -> [IfVeSMSuSecRwRtStLgrstOtwdInwdPos]
  IfVeSMSuSecRwRtStLgrstUpwdDnwdPos_Val_read/1 -> [IfVeSMSuSecRwRtStLgrstUpwdDnwdPos]
  IfVeSMSuSecRwRtStBkReclnUpwdDnwdPos_Val_read/1 -> [IfVeSMSuSecRwRtStBkReclnUpwdDnwdPos]
  IfVeSMSuSecRwRtStZeroPos_Val_read/1 -> [IfVeSMSuSecRwRtStZeroPos]
  Md57R2RZeroTrgtPosCalib_TrgtPosArray_read/1 -> Demux/1
  Demux/1 -> [VIPRMdR2RZeroTrgtPos]
  Demux/2 -> Terminator/1
  Demux/3 -> Terminator1/1
  Demux1/3 -> Terminator3/1
  Demux1/2 -> Terminator2/1
  Demux1/1 -> [VIPRR2RLgrstUpwdDnwdTrgtPos]
  Md57R2RLgrstUpwdDnwdTrgtPosCalib_TrgtPosArray_read/1 -> Demux1/1
  Md57R2RLgrstInwdOtwdTrgtPosCalib_TrgtPosArray_read/1 -> Demux2/1
  Demux2/1 -> [VIPRR2RLgrstInwdOtwdTrgtPos]
  Demux2/2 -> Terminator4/1
  Demux2/3 -> Terminator5/1
  Demux3/3 -> Terminator7/1
  Demux3/2 -> Terminator6/1
  Demux3/1 -> [VIPRR2RFwdBkwdTrgtPos]
  Md57R2RFwdBkwdTrgtPosCalib_TrgtPosArray_read/1 -> Demux3/1
  Md57R2RBkReclnUpwdDnwdTrgtPosCalib_TrgtPosArray_read/1 -> Demux4/1
  Demux4/1 -> [VIPRR2RBkReclnUpwdDnwdTrgtPos]
  Demux4/2 -> Terminator8/1
  Demux4/3 -> Terminator9/1
  Demux5/2 -> Terminator11/1
  Demux5/1 -> [Md57PassStCshnFldTrgtPos1]
  Md57PassStCshnFldTrgtPosCalib1_TrgtPosArray_read/1 -> Demux5/1
  Md57PassStFwdBkwdTrgtPosCalib1_TrgtPosArray_read/1 -> Demux6/1
  Demux6/1 -> [Md57PassStFwdBkwdTrgtPos1]
  Demux6/2 -> Terminator12/1
  IfVeSMSuPassStFldUpwdDnwdPos_Val_read/1 -> [IfVeSMSuPassStFldUpwdDnwdPos]
  [Md57PassStFwdBkwdTrgtPos1] -> Chart/25(PassStFwdBkwdTrgtPos1)
  [Md57PassStCshnFldTrgtPos1] -> Chart/27(PassStCshnFldTrgtPos1)
  [IfVeSMSuPassStFldUpwdDnwdPos] -> Chart/28(PassStFldUpwdDnwdPos)
  [PassStFwdBkwdPos] -> Chart/29(PassStFwdBkwdPos)
  Chart/14(FwdBkwdFailflg) -> [FwdBkwdFailflg]
  Chart/15(CshnFldFailflg) -> [CshnFldFailflg]
  If12/2 -> If Action Subsystem23/Action
  If12/1 -> If Action Subsystem24/Action
  Chart/13(PassStFldEn) -> If12/1
  PA_KeSMSuFirstRwStFwdBkwdPosDelta_Val/1 -> Chart/26(KeSMSuFirstRwStFwdBkwdPosDelta)
  Demux5/3 -> Terminator_18/1
  Demux6/3 -> Terminator_19/1
  [FwdBkwdFailflg] -> Unit Delay1/1
  [CshnFldFailflg] -> Unit Delay2/1
  IfVeSMSuPassStFrwdBkwdPos_Val_read/1 -> [PassStFwdBkwdPos]
  [PassStFldStgDone] -> Chart/30(PassStFldStgDone)
  Unit Delay1/1 -> Logical Operator7/3
  Unit Delay2/1 -> Logical Operator7/4
  [PassStBkReclnStgDone] -> Logical Operator3/1
  [PassStFldStgDone] -> Logical Operator3/2
  Logical Operator3/1 -> [PassStBkDone], Md57PassStBkStgDone_Val_write/1
  [PassStBkDone] -> Logical Operator5/1
  Logical Operator6/1 -> Logical Operator8/3
  [ThdRwLtStBkReclnStgDone] -> Logical Operator6/2
  [Is6s] -> Logical Operator6/1
  Logical Operator15/1 -> Logical Operator8/4
  [ThdRwLtStFwdBkwdStgDone] -> Logical Operator15/2
  [Is6s] -> Logical Operator15/1

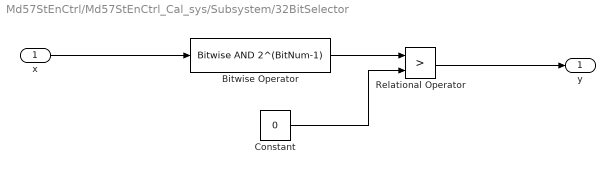
== system Md57StEnCtrl/Md57StEnCtrl_Cal_sys/Subsystem/32BitSelector ==
  x : Inport
  Bitwise Operator : simulink/Logic and Bit Operations/Bitwise Operator  logicop=AND  UseBitMask=on  BitMask=2^(BitNum-1)  BitMaskRealWorld=Stored Integer
  Constant : Constant  Value=0  OutDataTypeStr=uint32
  Relational Operator : RelationalOperator  Operator=>  OutDataTypeStr=boolean  RndMeth=Simplest
  y : Outport
  wires:
  Relational Operator/1 -> y/1
  Constant/1 -> Relational Operator/2
  x/1 -> Bitwise Operator/1
  Bitwise Operator/1 -> Relational Operator/1

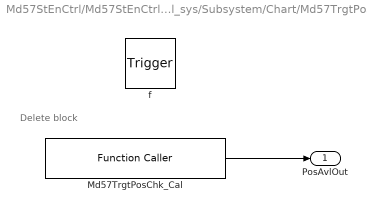
== system Md57StEnCtrl/Md57StEnCtrl_Cal_sys/Subsystem/Chart/Md57TrgtPosChk ==
  note: Delete block
  f : TriggerPort  TriggerType=function-call  VariantControl=(inherit)
      settings: CopyFcn=Stateflow.SLINSF.SimulinkMan.removeBlockPreDeleteFcn  PreDeleteFcn=Stateflow.SLINSF.SimulinkMan.unsafePredeleteFcn
  Md57TrgtPosChk_Cal : FunctionCaller  FunctionPrototype=PosAvl = Md57TrgtPosChk_Cal()  OutputArgumentSpecifications=uint8(1)
  PosAvlOut : Outport
  wires:
  Md57TrgtPosChk_Cal/1 -> PosAvlOut/1

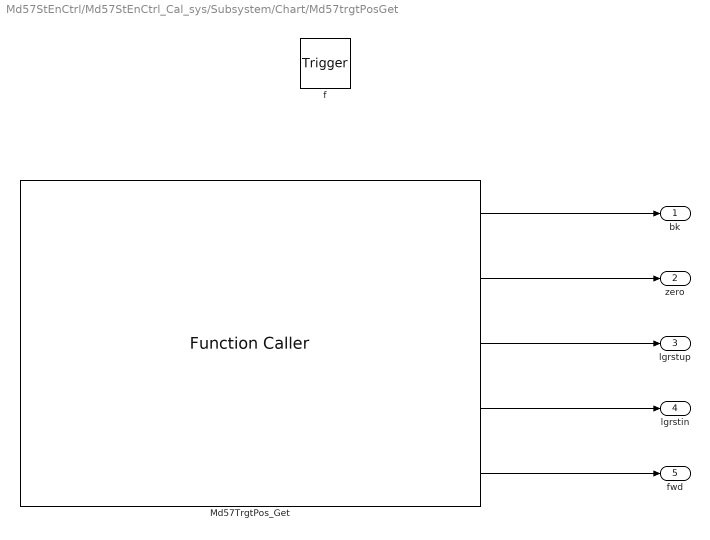
== system Md57StEnCtrl/Md57StEnCtrl_Cal_sys/Subsystem/Chart/Md57trgtPosGet ==
  f : TriggerPort  TriggerType=function-call  VariantControl=(inherit)
      settings: CopyFcn=Stateflow.SLINSF.SimulinkMan.removeBlockPreDeleteFcn  PreDeleteFcn=Stateflow.SLINSF.SimulinkMan.unsafePredeleteFcn
  Md57TrgtPos_Get : FunctionCaller  FunctionPrototype=[SecRwLtStBkReclnTrgtPos,SecRwLtStZeroTrgtPos,SecRwLtStLgrstUpwdDnwdTrgtPos,SecRwLtStLgrstInwdOtwdTrgtPos,SecRwLtStFwdBkwdTrgtPos] = Md57TrgtPos_Get()  OutputArgumentSpecifications=uint16(1), uint16(1), uint16(1), uint16(1), uint16(1)
  bk : Outport
  zero : Outport  Port=2
  lgrstup : Outport  Port=3
  lgrstin : Outport  Port=4
  fwd : Outport  Port=5
  wires:
  Md57TrgtPos_Get/1 -> bk/1
  Md57TrgtPos_Get/3 -> lgrstup/1
  Md57TrgtPos_Get/2 -> zero/1
  Md57TrgtPos_Get/4 -> lgrstin/1
  Md57TrgtPos_Get/5 -> fwd/1

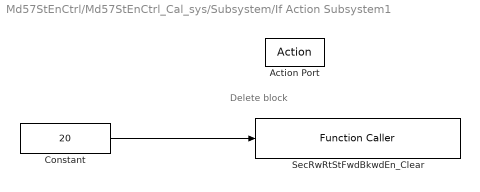
== system Md57StEnCtrl/Md57StEnCtrl_Cal_sys/Subsystem/If Action Subsystem1 ==
  note: Delete block
  Action Port : ActionPort  ActionType=else
  Constant : Constant  Value=20  OutDataTypeStr=uint8
  SecRwRtStFwdBkwdEn_Clear : FunctionCaller  FunctionPrototype=SecRwRtStFwdBkwdEn_Clear(data)  InputArgumentSpecifications=uint8(1)
  wires:
  Constant/1 -> SecRwRtStFwdBkwdEn_Clear/1

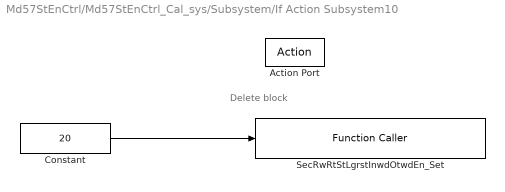
== system Md57StEnCtrl/Md57StEnCtrl_Cal_sys/Subsystem/If Action Subsystem10 ==
  note: Delete block
  Action Port : ActionPort  ActionType=then
  Constant : Constant  Value=20  OutDataTypeStr=uint8
  SecRwRtStLgrstInwdOtwdEn_Set : FunctionCaller  FunctionPrototype=SecRwRtStLgrstInwdOtwdEn_Set(data)  InputArgumentSpecifications=uint8(1)
  wires:
  Constant/1 -> SecRwRtStLgrstInwdOtwdEn_Set/1

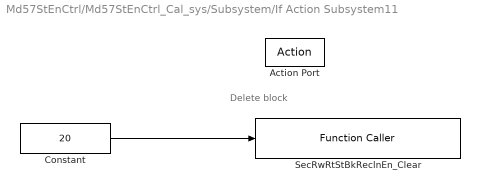
== system Md57StEnCtrl/Md57StEnCtrl_Cal_sys/Subsystem/If Action Subsystem11 ==
  note: Delete block
  Action Port : ActionPort  ActionType=else
  Constant : Constant  Value=20  OutDataTypeStr=uint8
  SecRwRtStBkReclnEn_Clear : FunctionCaller  FunctionPrototype=SecRwRtStBkReclnEn_Clear(data)  InputArgumentSpecifications=uint8(1)
  wires:
  Constant/1 -> SecRwRtStBkReclnEn_Clear/1

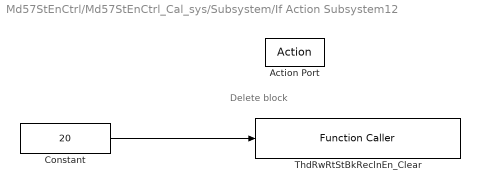
== system Md57StEnCtrl/Md57StEnCtrl_Cal_sys/Subsystem/If Action Subsystem12 ==
  note: Delete block
  Action Port : ActionPort  ActionType=else
  Constant : Constant  Value=20  OutDataTypeStr=uint8
  ThdRwRtStBkReclnEn_Clear : FunctionCaller  FunctionPrototype=ThdRwRtStBkReclnEn_Clear(data)  InputArgumentSpecifications=uint8(1)
  wires:
  Constant/1 -> ThdRwRtStBkReclnEn_Clear/1

== system Md57StEnCtrl/Md57StEnCtrl_Cal_sys/Subsystem/If Action Subsystem13 ==
  note: Delete block
  Action Port : ActionPort  ActionType=then
  Constant : Constant  Value=20  OutDataTypeStr=uint8
  ThdRwRtStBkReclnEn_Set : FunctionCaller  FunctionPrototype=ThdRwRtStBkReclnEn_Set(data)  InputArgumentSpecifications=uint8(1)
  wires:
  Constant/1 -> ThdRwRtStBkReclnEn_Set/1

== system Md57StEnCtrl/Md57StEnCtrl_Cal_sys/Subsystem/If Action Subsystem14 ==
  note: Delete block
  Action Port : ActionPort  ActionType=then
  Constant : Constant  Value=20  OutDataTypeStr=uint8
  SecRwRtStBkReclnEn_Set : FunctionCaller  FunctionPrototype=SecRwRtStBkReclnEn_Set(data)  InputArgumentSpecifications=uint8(1)
  wires:
  Constant/1 -> SecRwRtStBkReclnEn_Set/1

== system Md57StEnCtrl/Md57StEnCtrl_Cal_sys/Subsystem/If Action Subsystem15 ==
  note: Delete block
  Action Port : ActionPort  ActionType=else
  Constant : Constant  Value=20  OutDataTypeStr=uint8
  ThdRwRtStFwdBkwdEn_Clear : FunctionCaller  FunctionPrototype=ThdRwRtStFwdBkwdEn_Clear(data)  InputArgumentSpecifications=uint8(1)
  wires:
  Constant/1 -> ThdRwRtStFwdBkwdEn_Clear/1

== system Md57StEnCtrl/Md57StEnCtrl_Cal_sys/Subsystem/If Action Subsystem16 ==
  note: Delete block
  Action Port : ActionPort  ActionType=then
  Constant : Constant  Value=20  OutDataTypeStr=uint8
  ThdRwRtStFwdBkwdEn_Set : FunctionCaller  FunctionPrototype=ThdRwRtStFwdBkwdEn_Set(data)  InputArgumentSpecifications=uint8(1)
  wires:
  Constant/1 -> ThdRwRtStFwdBkwdEn_Set/1

== system Md57StEnCtrl/Md57StEnCtrl_Cal_sys/Subsystem/If Action Subsystem17 ==
  note: Delete block
  Action Port : ActionPort  ActionType=else
  Constant : Constant  Value=20  OutDataTypeStr=uint8
  PassStBkReclnEn_Clear : FunctionCaller  FunctionPrototype=PassStBkReclnEn_Clear(data)  InputArgumentSpecifications=uint8(1)
  wires:
  Constant/1 -> PassStBkReclnEn_Clear/1

== system Md57StEnCtrl/Md57StEnCtrl_Cal_sys/Subsystem/If Action Subsystem18 ==
  note: Delete block
  Action Port : ActionPort  ActionType=then
  Constant : Constant  Value=20  OutDataTypeStr=uint8
  PassStBkReclnEn_Set : FunctionCaller  FunctionPrototype=PassStBkReclnEn_Set(data)  InputArgumentSpecifications=uint8(1)
  wires:
  Constant/1 -> PassStBkReclnEn_Set/1

== system Md57StEnCtrl/Md57StEnCtrl_Cal_sys/Subsystem/If Action Subsystem19 ==
  note: Delete block
  Action Port : ActionPort  ActionType=else
  Constant : Constant  Value=20  OutDataTypeStr=uint8
  PassStFwdBkwdEn_Clear : FunctionCaller  FunctionPrototype=PassStFwdBkwdEn_Clear(data)  InputArgumentSpecifications=uint8(1)
  wires:
  Constant/1 -> PassStFwdBkwdEn_Clear/1

== system Md57StEnCtrl/Md57StEnCtrl_Cal_sys/Subsystem/If Action Subsystem2 ==
  note: Delete block
  Action Port : ActionPort  ActionType=then
  Constant : Constant  Value=20  OutDataTypeStr=uint8
  SecRwRtStFwdBkwdEn_Set : FunctionCaller  FunctionPrototype=SecRwRtStFwdBkwdEn_Set(data)  InputArgumentSpecifications=uint8(1)
  wires:
  Constant/1 -> SecRwRtStFwdBkwdEn_Set/1

== system Md57StEnCtrl/Md57StEnCtrl_Cal_sys/Subsystem/If Action Subsystem20 ==
  note: Delete block
  Action Port : ActionPort  ActionType=then
  Constant : Constant  Value=20  OutDataTypeStr=uint8
  PassStFwdBkwdEn_Set : FunctionCaller  FunctionPrototype=PassStFwdBkwdEn_Set(data)  InputArgumentSpecifications=uint8(1)
  wires:
  Constant/1 -> PassStFwdBkwdEn_Set/1

== system Md57StEnCtrl/Md57StEnCtrl_Cal_sys/Subsystem/If Action Subsystem21 ==
  note: Delete block
  Action Port : ActionPort  ActionType=else
  Constant : Constant  Value=20  OutDataTypeStr=uint8
  ZeroREn_Clear : FunctionCaller  FunctionPrototype=ZeroREn_Clear(data)  InputArgumentSpecifications=uint8(1)
  wires:
  Constant/1 -> ZeroREn_Clear/1

== system Md57StEnCtrl/Md57StEnCtrl_Cal_sys/Subsystem/If Action Subsystem22 ==
  note: Delete block
  Action Port : ActionPort  ActionType=then
  Constant : Constant  Value=20  OutDataTypeStr=uint8
  ZeroREn_Set : FunctionCaller  FunctionPrototype=ZeroREn_Set(data)  InputArgumentSpecifications=uint8(1)
  wires:
  Constant/1 -> ZeroREn_Set/1

== system Md57StEnCtrl/Md57StEnCtrl_Cal_sys/Subsystem/If Action Subsystem23 ==
  Action Port : ActionPort  ActionType=else
  Constant : Constant  Value=20  OutDataTypeStr=uint8
  PassStFldEn_Clear : FunctionCaller  FunctionPrototype=PassStFldEn_Clear(data)  InputArgumentSpecifications=uint8(1)
  wires:
  Constant/1 -> PassStFldEn_Clear/1

== system Md57StEnCtrl/Md57StEnCtrl_Cal_sys/Subsystem/If Action Subsystem24 ==
  Action Port : ActionPort  ActionType=then
  Constant : Constant  Value=20  OutDataTypeStr=uint8
  PassStFldEn_Set : FunctionCaller  FunctionPrototype=PassStFldEn_Set(data)  InputArgumentSpecifications=uint8(1)
  wires:
  Constant/1 -> PassStFldEn_Set/1

== system Md57StEnCtrl/Md57StEnCtrl_Cal_sys/Subsystem/If Action Subsystem3 ==
  note: Delete block
  note: Delete block
  note: Delete block
  Action Port : ActionPort  ActionType=else
  Constant : Constant  Value=20  OutDataTypeStr=uint8
  ThdRwLtStBkReclnEn_Clear : FunctionCaller  FunctionPrototype=ThdRwLtStBkReclnEn_Clear(data)  InputArgumentSpecifications=uint8(1)
  wires:
  Constant/1 -> ThdRwLtStBkReclnEn_Clear/1

== system Md57StEnCtrl/Md57StEnCtrl_Cal_sys/Subsystem/If Action Subsystem4 ==
  note: Delete block
  note: Delete block
  note: Delete block
  Action Port : ActionPort  ActionType=then
  Constant : Constant  Value=20  OutDataTypeStr=uint8
  ThdRwLtStBkReclnEn_Set : FunctionCaller  FunctionPrototype=ThdRwLtStBkReclnEn_Set(data)  InputArgumentSpecifications=uint8(1)
  wires:
  Constant/1 -> ThdRwLtStBkReclnEn_Set/1

== system Md57StEnCtrl/Md57StEnCtrl_Cal_sys/Subsystem/If Action Subsystem5 ==
  note: Delete block
  note: Delete block
  note: Delete block
  Action Port : ActionPort  ActionType=else
  Constant : Constant  Value=20  OutDataTypeStr=uint8
  ThdRwLtStFwdBkwdEn_Clear : FunctionCaller  FunctionPrototype=ThdRwLtStFwdBkwdEn_Clear(data)  InputArgumentSpecifications=uint8(1)
  wires:
  Constant/1 -> ThdRwLtStFwdBkwdEn_Clear/1

== system Md57StEnCtrl/Md57StEnCtrl_Cal_sys/Subsystem/If Action Subsystem6 ==
  note: Delete block
  note: Delete block
  note: Delete block
  Action Port : ActionPort  ActionType=then
  Constant : Constant  Value=20  OutDataTypeStr=uint8
  ThdRwLtStFwdBkwdEn_Set : FunctionCaller  FunctionPrototype=ThdRwLtStFwdBkwdEn_Set(data)  InputArgumentSpecifications=uint8(1)
  wires:
  Constant/1 -> ThdRwLtStFwdBkwdEn_Set/1

== system Md57StEnCtrl/Md57StEnCtrl_Cal_sys/Subsystem/If Action Subsystem7 ==
  note: Delete block
  Action Port : ActionPort  ActionType=else
  Constant : Constant  Value=20  OutDataTypeStr=uint8
  SecRwRtStLgrstUpwdDnwdEn_Clear : FunctionCaller  FunctionPrototype=SecRwRtStLgrstUpwdDnwdEn_Clear(data)  InputArgumentSpecifications=uint8(1)
  wires:
  Constant/1 -> SecRwRtStLgrstUpwdDnwdEn_Clear/1

== system Md57StEnCtrl/Md57StEnCtrl_Cal_sys/Subsystem/If Action Subsystem8 ==
  note: Delete block
  Action Port : ActionPort  ActionType=then
  Constant : Constant  Value=20  OutDataTypeStr=uint8
  SecRwRtStLgrstUpwdDnwdEn_Set : FunctionCaller  FunctionPrototype=SecRwRtStLgrstUpwdDnwdEn_Set(data)  InputArgumentSpecifications=uint8(1)
  wires:
  Constant/1 -> SecRwRtStLgrstUpwdDnwdEn_Set/1

== system Md57StEnCtrl/Md57StEnCtrl_Cal_sys/Subsystem/If Action Subsystem9 ==
  note: Delete block
  Action Port : ActionPort  ActionType=else
  Constant : Constant  Value=20  OutDataTypeStr=uint8
  SecRwRtStLgrstInwdOtwdEn_Clear : FunctionCaller  FunctionPrototype=SecRwRtStLgrstInwdOtwdEn_Clear(data)  InputArgumentSpecifications=uint8(1)
  wires:
  Constant/1 -> SecRwRtStLgrstInwdOtwdEn_Clear/1

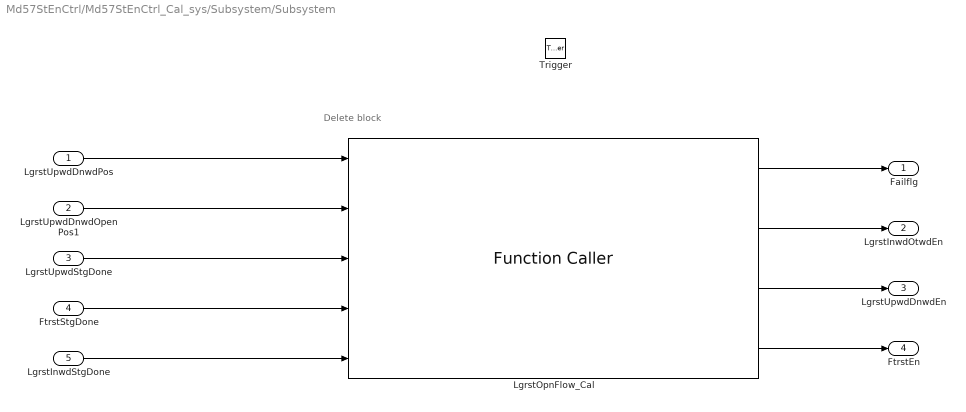
== system Md57StEnCtrl/Md57StEnCtrl_Cal_sys/Subsystem/Subsystem ==
  note: Delete block
  LgrstUpwdDnwdPos : Inport
  LgrstUpwdDnwdOpenPos1 : Inport  Port=2
  LgrstUpwdStgDone : Inport  Port=3
  FtrstStgDone : Inport  Port=4
  LgrstInwdStgDone : Inport  Port=5
  Trigger : TriggerPort  TriggerType=function-call  VariantControl=Variant  PortDimensions=1
  LgrstOpnFlow_Cal : FunctionCaller  FunctionPrototype=[Failflg,LgrstInwdOtwdEn,LgrstUpwdDnwdEn,FtrstEn] = LgrstOpnFlow_Cal(LgrstUpwdDnwdPos,LgrstUpwdDnwdOpenPos1,LgrstUpwdStgDone,FtrstStgDone,LgrstInwdStgDone)  InputArgumentSpecifications=uint16(1), uint16(1), boolean(true), boolean(true), boolean(true)  OutputArgumentSpecifications=boolean(true), boolean(true), boolean(true), boolean(true)
  Failflg : Outport
  LgrstInwdOtwdEn : Outport  Port=2
  LgrstUpwdDnwdEn : Outport  Port=3
  FtrstEn : Outport  Port=4
  wires:
  LgrstOpnFlow_Cal/2 -> LgrstInwdOtwdEn/1
  LgrstUpwdDnwdPos/1 -> LgrstOpnFlow_Cal/1
  LgrstOpnFlow_Cal/3 -> LgrstUpwdDnwdEn/1
  FtrstStgDone/1 -> LgrstOpnFlow_Cal/4
  LgrstUpwdStgDone/1 -> LgrstOpnFlow_Cal/3
  LgrstOpnFlow_Cal/4 -> FtrstEn/1
  LgrstInwdStgDone/1 -> LgrstOpnFlow_Cal/5
  LgrstUpwdDnwdOpenPos1/1 -> LgrstOpnFlow_Cal/2
  LgrstOpnFlow_Cal/1 -> Failflg/1
